simulink model "DHNV812163_genericExample"  (R2022b)
settings: Solver=VariableStepAuto  StartTime=0.0  StopTime=inf  RelTol=1e-3
undefined symbols (not defined in the file or in its folder): h_max, heatMax, P_h
libraries: rllib x1
settings Model: Creator=ditle  LastModifiedBy=ditle
settings OptimizationCC: BlockReduction=off  DefaultParameterBehavior=Inlined  BufferReuse=off

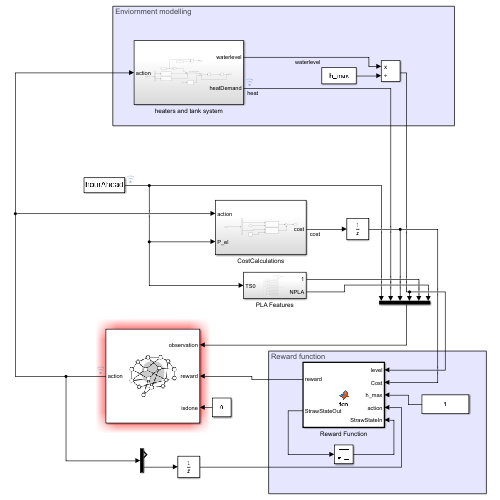
[thumbnail: Simulink's stored preview of the top-level diagram]
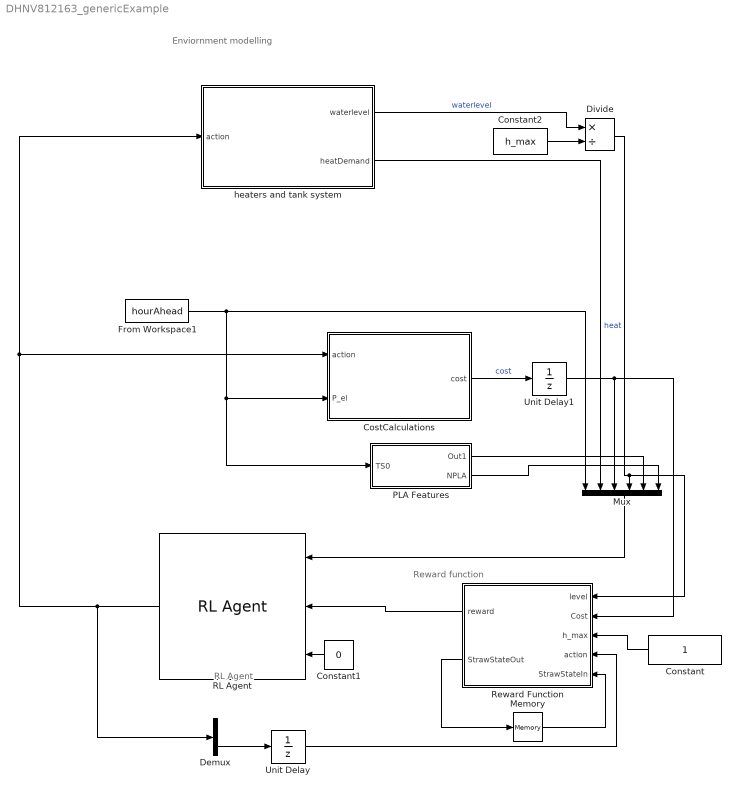
== system DHNV812163_genericExample ==
  note: Reward function
  note: Enviornment modelling
  note: RL Agent
  Constant : Constant
  Constant1 : Constant  Value=0
  Constant2 : Constant  Value=h_max
  CostCalculations : Subsystem
  Demux : Demux  Outputs=2
  Divide : Product  Inputs=*/  RndMeth=Zero  SaturateOnIntegerOverflow=on
  From Workspace1 : FromWorkspace  VariableName=hourAhead  SampleTime=1
  Memory : Memory
  Mux : Mux  Inputs=6
  PLA Features : Subsystem
  RL Agent : rllib/RL Agent  Agent=agentObj  ExternalActionAsInput=off  ProvideLastAction=off  ProvideCumRwd=off  TreatAsDirectFeedthrough=on  UseStrictObservationDataTypes=off
  Reward Function : MATLAB Function  TreatAsAtomicUnit=on  SystemSampleTime=1
  Unit Delay : UnitDelay  SampleTime=-1  HasFrameUpgradeWarning=on
  Unit Delay1 : UnitDelay  SampleTime=-1  HasFrameUpgradeWarning=on
  heaters and tank system : Subsystem
  wires:
  From Workspace1/1 -> Mux/1, PLA Features/1(TS0), CostCalculations/2(P_el)
  Unit Delay1/1 -> Reward Function/2(Cost), Mux/3
  RL Agent/1 -> CostCalculations/1(action), heaters and tank system/1(action), Demux/1
  heaters and tank system/1(waterlevel) -> Divide/1  "waterlevel"
  Mux/1 -> RL Agent/1
  Constant1/1 -> RL Agent/3
  Constant/1 -> Reward Function/3(h_max)
  Reward Function/1(reward) -> RL Agent/2
  Divide/1 -> Reward Function/1(level), Mux/4
  Constant2/1 -> Divide/2
  CostCalculations/1(cost) -> Unit Delay1/1  "cost"
  PLA Features/1(Out1) -> Mux/5
  PLA Features/2(NPLA) -> Mux/6
  Demux/2 -> Unit Delay/1
  Reward Function/2(StrawStateOut) -> Memory/1
  Memory/1 -> Reward Function/5(StrawStateIn)
  Unit Delay/1 -> Reward Function/4(action)
  heaters and tank system/2(heatDemand) -> Mux/2  "heat"

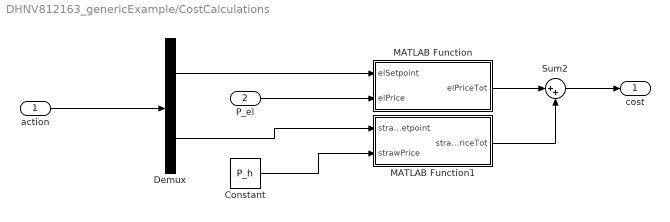
== system DHNV812163_genericExample/CostCalculations ==
  action : Inport
  P_el : Inport  Port=2
  Constant : Constant  Value=P_h
  Demux : Demux  Outputs=2
  MATLAB Function : MATLAB Function  TreatAsAtomicUnit=on
  MATLAB Function1 : MATLAB Function  TreatAsAtomicUnit=on
  Sum2 : Sum  Inputs=|++
  cost : Outport
  wires:
  action/1 -> Demux/1
  P_el/1 -> MATLAB Function/2(elPrice)
  Constant/1 -> MATLAB Function1/2(strawPrice)
  Demux/2 -> MATLAB Function1/1(strawSetpoint)
  MATLAB Function/1(elPriceTot) -> Sum2/1
  MATLAB Function1/1(strawPriceTot) -> Sum2/2
  Demux/1 -> MATLAB Function/1(elSetpoint)
  Sum2/1 -> cost/1

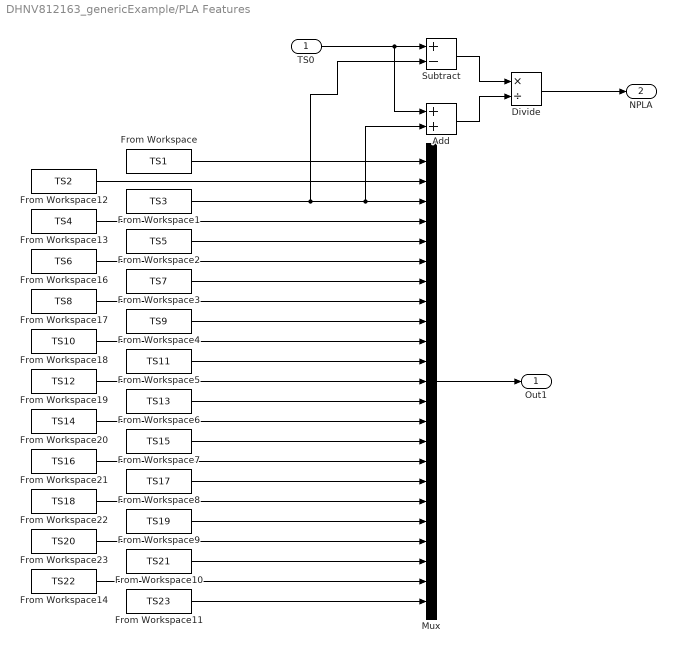
== system DHNV812163_genericExample/PLA Features ==
  TS0 : Inport
  Add : Sum
  Divide : Product  Inputs=*/  RndMeth=Zero  SaturateOnIntegerOverflow=on
  From Workspace : FromWorkspace  VariableName=TS1
  From Workspace1 : FromWorkspace  VariableName=TS3
  From Workspace10 : FromWorkspace  VariableName=TS21
  From Workspace11 : FromWorkspace  VariableName=TS23
  From Workspace12 : FromWorkspace  VariableName=TS2
  From Workspace13 : FromWorkspace  VariableName=TS4
  From Workspace14 : FromWorkspace  VariableName=TS22
  From Workspace16 : FromWorkspace  VariableName=TS6
  From Workspace17 : FromWorkspace  VariableName=TS8
  From Workspace18 : FromWorkspace  VariableName=TS10
  From Workspace19 : FromWorkspace  VariableName=TS12
  From Workspace2 : FromWorkspace  VariableName=TS5
  From Workspace20 : FromWorkspace  VariableName=TS14
  From Workspace21 : FromWorkspace  VariableName=TS16
  From Workspace22 : FromWorkspace  VariableName=TS18
  From Workspace23 : FromWorkspace  VariableName=TS20
  From Workspace3 : FromWorkspace  VariableName=TS7
  From Workspace4 : FromWorkspace  VariableName=TS9
  From Workspace5 : FromWorkspace  VariableName=TS11
  From Workspace6 : FromWorkspace  VariableName=TS13
  From Workspace7 : FromWorkspace  VariableName=TS15
  From Workspace8 : FromWorkspace  VariableName=TS17
  From Workspace9 : FromWorkspace  VariableName=TS19
  Mux : Mux  Inputs=23
  Subtract : Sum  Inputs=+-
  Out1 : Outport
  NPLA : Outport  Port=2
  wires:
  Mux/1 -> Out1/1
  From Workspace/1 -> Mux/1
  From Workspace1/1 -> Subtract/2, Add/2, Mux/3
  From Workspace2/1 -> Mux/5
  From Workspace5/1 -> Mux/11
  From Workspace4/1 -> Mux/9
  From Workspace3/1 -> Mux/7
  From Workspace11/1 -> Mux/23
  From Workspace10/1 -> Mux/21
  From Workspace9/1 -> Mux/19
  From Workspace8/1 -> Mux/17
  From Workspace7/1 -> Mux/15
  From Workspace6/1 -> Mux/13
  From Workspace12/1 -> Mux/2
  From Workspace13/1 -> Mux/4
  From Workspace16/1 -> Mux/6
  From Workspace18/1 -> Mux/10
  From Workspace17/1 -> Mux/8
  From Workspace19/1 -> Mux/12
  From Workspace20/1 -> Mux/14
  From Workspace21/1 -> Mux/16
  From Workspace22/1 -> Mux/18
  From Workspace23/1 -> Mux/20
  From Workspace14/1 -> Mux/22
  TS0/1 -> Add/1, Subtract/1
  Subtract/1 -> Divide/1
  Add/1 -> Divide/2
  Divide/1 -> NPLA/1

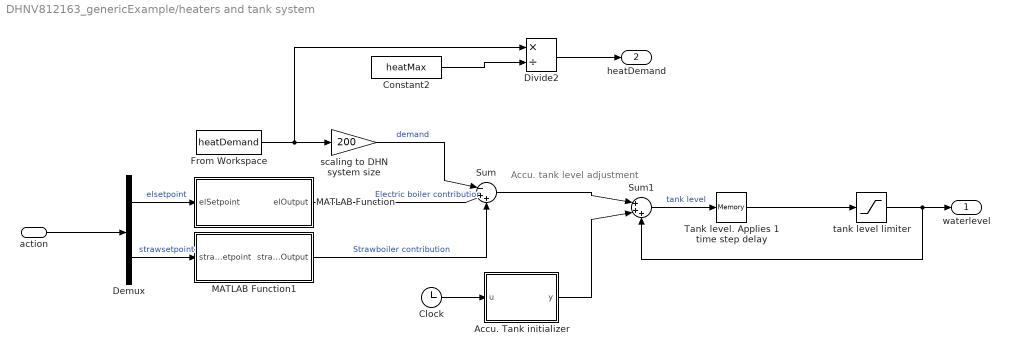
== system DHNV812163_genericExample/heaters and tank system ==
  note: Accu. tank level adjustment
  action : Inport
  Accu. Tank initializer : MATLAB Function  TreatAsAtomicUnit=on
  Clock : Clock
  Constant2 : Constant  Value=heatMax
  Demux : Demux  Outputs=2
  Divide2 : Product  Inputs=*/  RndMeth=Zero  SaturateOnIntegerOverflow=on
  From Workspace : FromWorkspace  VariableName=heatDemand  SampleTime=1
  MATLAB Function : MATLAB Function  TreatAsAtomicUnit=on  SystemSampleTime=1
  MATLAB Function1 : MATLAB Function  TreatAsAtomicUnit=on  SystemSampleTime=1
  Sum : Sum  Inputs=|-++
  Sum1 : Sum  Inputs=|+++
  Tank level. Applies 1 time step delay : Memory  InheritSampleTime=on
  scaling to DHN system size : Gain  Gain=200
  tank level limiter : Saturate  UpperLimit=h_max  LowerLimit=0
  waterlevel : Outport
  heatDemand : Outport  Port=2
  wires:
  From Workspace/1 -> Divide2/1, scaling to DHN system size/1
  action/1 -> Demux/1
  Demux/1 -> MATLAB Function/1(elSetpoint)  "elsetpoint"
  Demux/2 -> MATLAB Function1/1(strawSetpoint)  "strawsetpoint"
  MATLAB Function/1(elOutput) -> Sum/2  "Electric boiler contribution"
  MATLAB Function1/1(strawOutput) -> Sum/3  "Strawboiler contribution"
  Sum/1 -> Sum1/1
  Sum1/1 -> Tank level. Applies 1 time step delay/1  "tank level"
  Clock/1 -> Accu. Tank initializer/1(u)
  Accu. Tank initializer/1(y) -> Sum1/2
  Tank level. Applies 1 time step delay/1 -> tank level limiter/1
  tank level limiter/1 -> Sum1/3, waterlevel/1
  Constant2/1 -> Divide2/2
  Divide2/1 -> heatDemand/1
  scaling to DHN system size/1 -> Sum/1  "demand"

== matlab function DHNV812163_genericExample/Reward Function ==
  data: level input; reward output; Cost input; h_max input; action input; StrawStateIn input; StrawStateOut output
function [reward, StrawStateOut] = fcn(level,Cost,h_max,action,StrawStateIn)


if (h_max*0.1 <= level) && (level <= h_max*0.9)
    r1 = -Cost; %-P
elseif (h_max*0.9 < level)
    r1 = -Cost-(level-h_max)^2-1;
else 
    r1 = -Cost-(h_max*0.1-level)^2-1;
end

if action == 1 && StrawStateIn == 0
    r2 = -0;
    StrawStateOut = 1;
elseif action ==0 && StrawStateIn == 1
    StrawStateOut = 0;
    r2 = 0;
else
    StrawStateOut = StrawStateIn;
    r2 = 0;
end


reward = r1 +r2;




%u start-up:
%if (h_max*0.1 <= level) && (level <= h_max*0.9)
%    r = -P; %-P
%elseif (h_max*0.9 < level)
%    r = -P-(level-h_max)^2-1;
%else 
%    r = -P-(h_max*0.1-level)^2-1;
%end


%if (h_max*0.1 <= level) && (level <= h_max*0.9)
%    r = -P;
%elseif (h_max*0.9 < level)
%    r = -P-(level-h_max*0.9)^2;
%elseif (h_max*0.1 > level) %0-10% penalty
%    r = -P-(h_max*0.1-level)^2;
%else
%    r = 1;
%end


%if (h_max*0.1 <= level) && (level <= h_max*0.95)
%    r = -P;
%else
%    r = -P-100000000000000; %(0.5*P*abs(level-h_max));
%end

== matlab function DHNV812163_genericExample/CostCalculations/MATLAB Function ==
  data: elSetpoint input; elPriceTot output; elPrice input
function elPriceTot = fcn(elSetpoint, elPrice)
 
switch int8(elSetpoint)
    case 0
        temp = 0;
    case 1
        temp = 0.347;
     otherwise
        error('Invalid input')
end

%switch int8(elSetpoint)
%    case 0
%        temp = 0;
%    case 1
%        temp = 600;
%    case 2
%        temp = 1200;
%    case 3
%        temp = 1800;
%    case 4
%        temp = 2400;
%    otherwise
%        error('Invalid input')
%end


elPriceTot = temp*elPrice;

== matlab function DHNV812163_genericExample/CostCalculations/MATLAB Function1 ==
  data: strawSetpoint input; strawPriceTot output; strawPrice input
function strawPriceTot = fcn(strawSetpoint, strawPrice)
 
switch int8(strawSetpoint)
    case 0
        temp = 0;
    case 1
        temp = 0.652;
    otherwise
        error('Invalid input')
end


%switch int8(strawSetpoint)
%    case 0
%        temp = 0;
%    case 1
%        temp = 1125;
%    case 2
%        temp = 2250;
%    case 3
%        temp = 3375;
%    case 4
%        temp = 4500;
%    otherwise
%        error('Invalid input')
%end

strawPriceTot = temp*strawPrice;

== matlab function DHNV812163_genericExample/heaters and tank system/MATLAB Function ==
  data: elSetpoint input; elOutput output
function elOutput = fcn(elSetpoint)
    
switch int8(elSetpoint)
    case 0
        elOutput = 0;
    case 1
        elOutput = 2400;
    otherwise
        error('Invalid input')
end

%switch int8(elSetpoint)
%    case 0
%        elOutput = 0;
%    case 1
%        elOutput = 600;
%    case 2
%        elOutput = 1200;
%    case 3
%        elOutput = 1800;
%    case 4
%        elOutput = 2400;
%    otherwise
%        error('Invalid input')
%end

== matlab function DHNV812163_genericExample/heaters and tank system/MATLAB Function1 ==
  data: strawSetpoint input; strawOutput output
function strawOutput = fcn(strawSetpoint)

switch int8(strawSetpoint)
    case 0
        strawOutput = 0;
    case 1
        strawOutput = 4500;
    otherwise
        error('Invalid input')
end


%switch int8(strawSetpoint)
%    case 0
%        strawOutput = 0;
%    case 1
%        strawOutput = 1125;
%    case 2
%        strawOutput = 2250;
%    case 3
%        strawOutput = 3375;
%    case 4
%        strawOutput = 4500;
%    otherwise
%        error('Invalid input')
%end

== matlab function DHNV812163_genericExample/heaters and tank system/Accu. Tank initializer ==
  data: u input; y output
function y = fcn(u)

if u == 0
    y = 40000;
else
   y = 0;
end
